simulink model "Noise_Effecr_on_Analog_Transmission"  (R2018a)
settings: Solver=VariableStepAuto  StartTime=0.0  StopTime=20.0  RelTol=1e-3
libraries: dsparch4 x3, dspmathops x2, dspsrcs4 x1
settings Model: Creator=ashwin  LastModifiedBy=ashwin

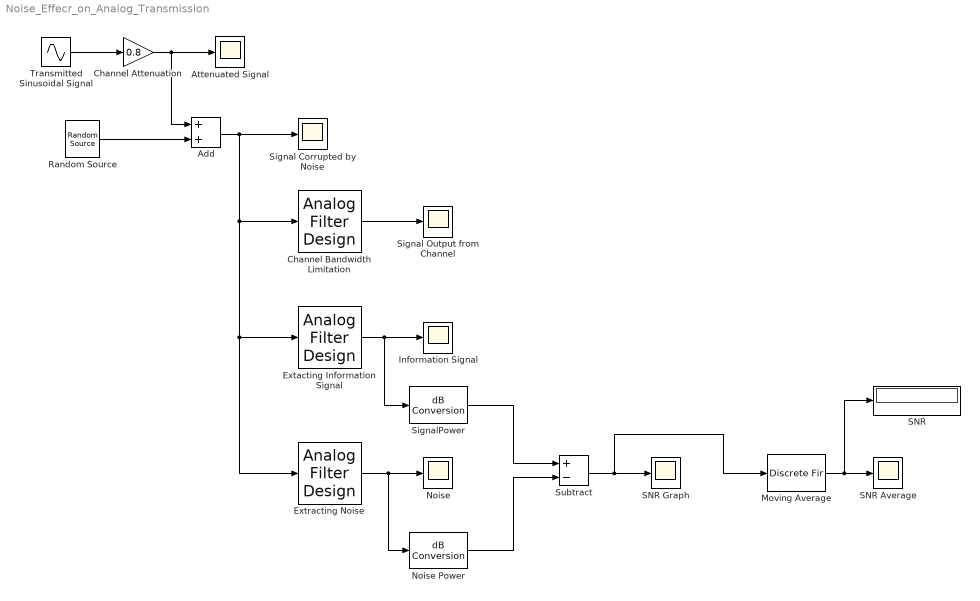
== system Noise_Effecr_on_Analog_Transmission ==
  Add : Sum
  Attenuated Signal : Scope
  Channel Attenuation : Gain  Gain=0.8
  Channel Bandwidth Limitation : dsparch4/Analog Filter Design  method=Butterworth  filttype=Lowpass  N=10  Wlo=1000  Whi=80  Rp=2  Rs=40
  Extacting Information Signal : dsparch4/Analog Filter Design  method=Butterworth  filttype=Bandpass  N=10  Wlo=195  Whi=205  Rp=2  Rs=40
  "Extracting Noise " : dsparch4/Analog Filter Design  method=Butterworth  filttype=Bandstop  N=10  Wlo=195  Whi=205  Rp=2  Rs=40
  Information Signal : Scope
  Moving Average : DiscreteFir  Coefficients=ones(1, 1000)/1000  SampleTime=0.001
  Noise : Scope
  "Noise Power " : dspmathops/dB Conversion  dBtype=dB  intype=Amplitude  R=1  fuzz=off
      settings: SourceProductName=DSP System Toolbox
  Random Source : dspsrcs4/Random Source  SrcType=Gaussian  NormMethod=Ziggurat  CltLength=12  MinVal=0  MaxVal=1  MeanVal=0  VarVal=1  RepMode=Not repeatable  rawSeed=1  IsInherit=off  SampMode=Discrete  SampTime=0.001  SampFrame=1  DataType=Double  OutComplex=Real  OutputFrames=off
  SNR : Display
  SNR Average : Scope
  SNR Graph : Scope
  Signal Output from Channel : Scope
  Signal Corrupted by Noise : Scope
  SignalPower : dspmathops/dB Conversion  dBtype=dB  intype=Amplitude  R=1  fuzz=off
      settings: SourceProductName=DSP System Toolbox
  Subtract : Sum  Inputs=+-
  Transmitted Sinusoidal Signal : Sin  Amplitude=10  Frequency=200  SampleTime=0.001
  wires:
  Transmitted Sinusoidal Signal/1 -> Channel Attenuation/1
  Channel Attenuation/1 -> Add/1, Attenuated Signal/1
  Random Source/1 -> Add/2
  Add/1 -> Signal Corrupted by Noise/1, Extacting Information Signal/1, "Extracting Noise "/1, Channel Bandwidth Limitation/1
  Channel Bandwidth Limitation/1 -> Signal Output from Channel/1
  Extacting Information Signal/1 -> Information Signal/1, SignalPower/1
  "Extracting Noise "/1 -> "Noise Power "/1, Noise/1
  "Noise Power "/1 -> Subtract/2
  SignalPower/1 -> Subtract/1
  Subtract/1 -> Moving Average/1, SNR Graph/1
  Moving Average/1 -> SNR/1, SNR Average/1
